simulink model "observer_simulacao_2014a"  (R2014a)
settings: Solver=ode4  StartTime=0.0  StopTime=300  FixedStep=0.1  RelTol=1e-3
settings Model: Creator=icaro  LastModifiedBy=MatheusWhite
settings DebuggingCC: MergeDetectMultiDrivingBlocksExec=error  FrameProcessingCompatibilityMsg=error

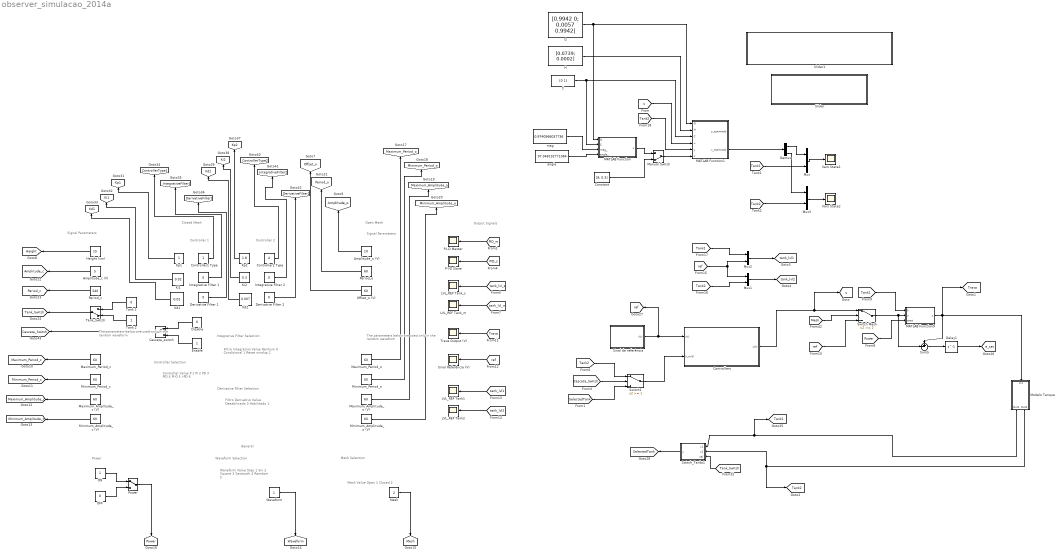
== system observer_simulacao_2014a ==
  note: Waveform Selection
  note: Mesh Selection
  note: Signal Parameters
  note: The parameters below are used only in the random waveform
  note: Filtro Integrativo
      | Value
      |
      | Nenhum
      | 0
      |
      | Condicional
      | 1
      |
      | Reset windup
      | 2
  note: Power
  note: Controller
      | Value
      |
      | P
      | 1
      |
      | PI
      | 2
      |
      | PD
      | 3
      |
      | PID
      | 4
      |
      | PI-D
      | 5
      |
      | I-PD
      | 6
  note: General
  note: Derivative Filter Selection
  note: Closed Mesh
  note: The parameters below are used only in the random waveform
  note: Signal Parameters
  note: Controller 2
  note: Mesh
      | Value
      |
      | Open
      | 1
      |
      | Closed
      | 2
  note: Filtro Derivativo
      | Value
      |
      | Desabilitado
      | 0
      |
      | Habilitado
      | 1
  note: Waveform
      | Value
      |
      | Step
      | 1
      |
      | Sin
      | 2
      |
      | Square
      | 3
      |
      | Sawtooth
      | 4
      |
      | Ramdom
      | 5
  note: Open Mesh
  note: Output Signals
  note: Integrative Filter Selection
  note: Controller 1
  note: Controller Selection
  Amplitude_c (V) : Constant  Value=5
  Amplitude_o (V) : Constant  Value=10
  C : Constant  Value=[0 1]  VectorParams1D=off
  Cascata_switch : ManualSwitch
  Constant : Constant  Value=[8; 0.3]
  Controller1 Type : Constant
  Controller2 Type : Constant  Value=4
  Controllers : Subsystem
  Delay1 : Delay  DelayLength=1  InitialCondition=0
  Demux : Demux  Outputs=2
  Derivative Filter 1 : Constant  Value=0
  Derivative Filter 2 : Constant  Value=0
  Disable : Constant  Value=0
  Enable : Constant
  G : Constant  Value=[0.9942 0; 0.0057 0.9942]  VectorParams1D=off
  H : Constant  Value=[0.0739; 0.0002]  VectorParams1D=off
  Height (cm) : Constant  Value=15
  Integrative Filter 1 : Constant  Value=0
  Integrative Filter 2 : Constant  Value=0
  Kd1 : Constant  Value=0.01
  Kd2 : Constant  Value=0.007
  Ki1 : Constant  Value=0.02
  Ki2 : Constant  Value=0.3
  Kp1 : Constant
  Kp2 : Constant  Value=1.8
  LVL_REF Tank1 : Scope
      settings: TimeRange=100  ShowLegends=on  MaxDataPoints=5000  SaveName=tank1level1  YMin=0  YMax=30  SampleTime=-1  DataFormat=Array
  LVL_REF Tank2 : Scope
      settings: TimeRange=250  ShowLegends=on  MaxDataPoints=5000  SaveName=tank2level1  YMin=0  YMax=30  SampleTime=-1  DataFormat=Array
  "LVL_REF Tank_m " : Scope
      settings: TimeRange=300  ShowLegends=on  MaxDataPoints=5000  SaveName=tank2level  YMin=0  YMax=30  SampleTime=-1  DataFormat=Array
  LVL_REF Tank_s : Scope
      settings: TimeRange=300  ShowLegends=on  MaxDataPoints=5000  SaveName=tank1level  YMin=-90  YMax=130  SampleTime=-1  DataFormat=Array
  MATLAB Function : MATLAB Function  TreatAsAtomicUnit=on
      settings: PermitHierarchicalResolution=ParametersOnly
  MATLAB Function1 : MATLAB Function  TreatAsAtomicUnit=on
      settings: PermitHierarchicalResolution=ParametersOnly
  MATLAB Function9 : MATLAB Function  TreatAsAtomicUnit=on
      settings: PermitHierarchicalResolution=ParametersOnly
  Manual Switch : ManualSwitch  CurrentSetting=0
  Maximum_Amplitude_c (V) : Constant  Value=60
  Maximum_Amplitude_o (V) : Constant  Value=60
  Maximum_Period_c : Constant  Value=60
  Maximum_Period_o : Constant  Value=60
  Mesh : Constant  Value=2
  Minimum_Amplitude_c (V) : Constant  Value=60
  Minimum_Amplitude_o (V) : Constant  Value=60
  Minimum_Period_c : Constant  Value=60
  Minimum_Period_o : Constant  Value=60
  Modelo Tanque : Subsystem
  Mux{,1..3} (4 alike) : Mux  Inputs=2
  OFF : Constant  Value=0
  ON : Constant
  Offset_o (V) : Constant  Value=60
  P-I-D Master : Scope
      settings: TimeRange=300  ShowLegends=on  MaxDataPoints=5000  SaveName=PID1  YMin=-35  YMax=30  SampleTime=-1  DataFormat=Array
  P-I-D Slave : Scope
      settings: TimeRange=300  ShowLegends=on  MaxDataPoints=5000  SaveName=PID2  YMin=-35  YMax=80  SampleTime=-1  DataFormat=Array
  Period_c : Constant  Value=240
  Period_o : Constant  Value=60
  Power : ManualSwitch
  Sinal Referência (V) : Scope
      settings: TimeRange=300  MaxDataPoints=5000  SaveName=meshoutput  YMin=0  YMax=30  SampleTime=-1  DataFormat=Array
  Sinal de referência : Subsystem
  Slider : Subsystem  Description=Replaced Block  mask(Replaced Block){}
      mask help: This block has been replaced with an empty subsystem because it used functionality that is unavailable in Simulink R2014a.
      mask Display: fprintf('Replaced: %s\n','Dashboard Widget')
  Slider1 : Subsystem  Description=Replaced Block  mask(Replaced Block){}
      mask help: This block has been replaced with an empty subsystem because it used functionality that is unavailable in Simulink R2014a.
      mask Display: fprintf('Replaced: %s\n','Dashboard Widget')
  Sum5 : Sum  Inputs=+-|
  Switch Mesh : Switch  Threshold=2
  Switch1 : Switch  Threshold=1
  Switch_Tanks1 : MATLAB Function  TreatAsAtomicUnit=on
      settings: PermitHierarchicalResolution=ParametersOnly
  Tank 1 : Constant  Value=0
  Tank 2 : Constant
  Tank_Switch : ManualSwitch  CurrentSetting=0
  Trava Output (V) : Scope
      settings: TimeRange=300  MaxDataPoints=5000  SaveName=meshoutput2  YMin=-4.5  YMax=4.5  SampleTime=-1  DataFormat=Array
  Vars State1 : Scope
      settings: TimeRange=300  ShowLegends=on  MaxDataPoints=5000  SaveToWorkspace=off  SaveName=ScopeData  YMin=-1.00000  YMax=30.00000  SampleTime=-1
  Vars State2 : Scope
      settings: TimeRange=300  ShowLegends=on  MaxDataPoints=5000  SaveToWorkspace=off  YMin=-1.85008  YMax=16.65074  SampleTime=-1
  Waveform : Constant
  angle : Constant  Value=97.048192771084
  mag : Constant  Value=0.9740566037736
  tag scope: Amplitude_c=global, Amplitude_o=global, Cascata_Switch=global, ControllerType1=global, ControllerType2=global, DerivativeFilter1=global, DerivativeFilter2=global, Height=global, IntegrativeFilter1=global, IntegrativeFilter2=global, Kd1=global, Kd2=global, Ki1=global, Ki2=global, Kp1=global, Kp2=global, Maximum_Amplitude_c=global, Maximum_Amplitude_o=global, Maximum_Period_c=global, Maximum_Period_o=global, Mesh=global, Minimum_Amplitude_c=global, Minimum_Amplitude_o=global, Minimum_Period_c=global, Minimum_Period_o=global, Offset_o=global, Period_c=global, Period_o=global, Power=global, SelectedTank=global, Tank1=global, Tank2=global, Tank_Switch=global, Trava=global, Waveform=global, e_sat=global, ref=global, tank_lvl1=global, tank_lvl2=global, u=global
  wires:
  Maximum_Period_o/1 -> [Maximum_Period_o]
  Integrative Filter 2/1 -> [IntegrativeFilter2]
  [Power] -> MATLAB Function9/3(start)
  MATLAB Function/1(L) -> Manual Switch/1
  Manual Switch/1 -> MATLAB Function1/6(L)
  Controller2 Type/1 -> [ControllerType2]
  [Tank1] -> Mux/2
  [tank_lvl_m] -> "LVL_REF Tank_m "/1
  Switch_Tanks1/1(y) -> [SelectedTank]
  [Tank2] -> MATLAB Function1/5(y)
  [ref] -> Mux2/2, Mux1/1
  Minimum_Amplitude_o (V)/1 -> [Minimum_Amplitude_o]
  [Tank2] -> Mux1/2
  Minimum_Period_o/1 -> [Minimum_Period_o]
  MATLAB Function1/2(x_estimado) -> Demux/1
  [Tank_Switch] -> Switch_Tanks1/3(sel)
  [tank_lvl2] -> LVL_REF Tank2/1
  Mux/1 -> Vars State1/1
  Amplitude_o (V)/1 -> [Amplitude_o]
  [PID_m] -> P-I-D Master/1
  Mux1/1 -> [tank_lvl2]
  Delay1/1 -> [e_sat]
  angle/1 -> MATLAB Function/4(angle_)
  mag/1 -> MATLAB Function/3(mag_)
  Power/1 -> [Power]
  [Trava] -> Trava Output (V)/1
  Disable/1 -> Cascata_switch/1
  [ref] -> Switch Mesh/3
  Kp2/1 -> [Kp2]
  [Tank1] -> MATLAB Function9/1(h)
  Controllers/1(u(t)) -> [u], Switch Mesh/1
  [Tank1] -> Mux2/1
  Sinal de referência/1(r(t)) -> Controllers/1(r(t)), [ref]
  Minimum_Amplitude_c (V)/1 -> [Minimum_Amplitude_c]
  [tank_lvl1] -> LVL_REF Tank1/1
  [Mesh] -> Switch Mesh/2
  Sum5/1 -> Delay1/1
  Modelo Tanque/1(Out1) -> Switch_Tanks1/1(x1), [Tank1]
  Derivative Filter 2/1 -> [DerivativeFilter2]
  Switch Mesh/1 -> Sum5/2, MATLAB Function9/2(u)
  Integrative Filter 1/1 -> [IntegrativeFilter1]
  Enable/1 -> Cascata_switch/2
  Cascata_switch/1 -> [Cascata_Switch]
  [u] -> MATLAB Function1/4(u)
  Controller1 Type/1 -> [ControllerType1]
  Period_o/1 -> [Period_o]
  [ref] -> Sinal Referência (V)/1
  Tank 1/1 -> Tank_Switch/1
  [Cascata_Switch] -> Switch1/2
  Kd2/1 -> [Kd2]
  Kd1/1 -> [Kd1]
  Ki2/1 -> [Ki2]
  Amplitude_c (V)/1 -> [Amplitude_c]
  Height (cm)/1 -> [Height]
  OFF/1 -> Power/2
  [tank_lvl_s] -> LVL_REF Tank_s/1
  [PID_s] -> P-I-D Slave/1
  [SelectedTank] -> Switch1/3
  Minimum_Period_c/1 -> [Minimum_Period_c]
  Period_c/1 -> [Period_c]
  Maximum_Period_c/1 -> [Maximum_Period_c]
  Tank 2/1 -> Tank_Switch/2
  Ki1/1 -> [Ki1]
  Maximum_Amplitude_o (V)/1 -> [Maximum_Amplitude_o]
  Offset_o (V)/1 -> [Offset_o]
  Waveform/1 -> [Waveform]
  Kp1/1 -> [Kp1]
  Constant/1 -> Manual Switch/2
  Maximum_Amplitude_c (V)/1 -> [Maximum_Amplitude_c]
  MATLAB Function9/1(y) -> Modelo Tanque/1(In1), [Trava], Sum5/1
  Tank_Switch/1 -> [Tank_Switch]
  Modelo Tanque/2(Out2) -> Switch_Tanks1/2(x2), [Tank2]
  [Tank2] -> Switch1/1
  Mux2/1 -> [tank_lvl1]
  Derivative Filter 1/1 -> [DerivativeFilter1]
  ON/1 -> Power/1
  Mesh/1 -> [Mesh]
  Switch1/1 -> Controllers/2(h_m(t))
  Demux/1 -> Mux/1
  Mux3/1 -> Vars State2/1
  [Tank2] -> Mux3/2
  Demux/2 -> Mux3/1
  C/1 -> MATLAB Function1/3(C), MATLAB Function/2(C)
  G/1 -> MATLAB Function1/1(G), MATLAB Function/1(G)
  H/1 -> MATLAB Function1/2(H)

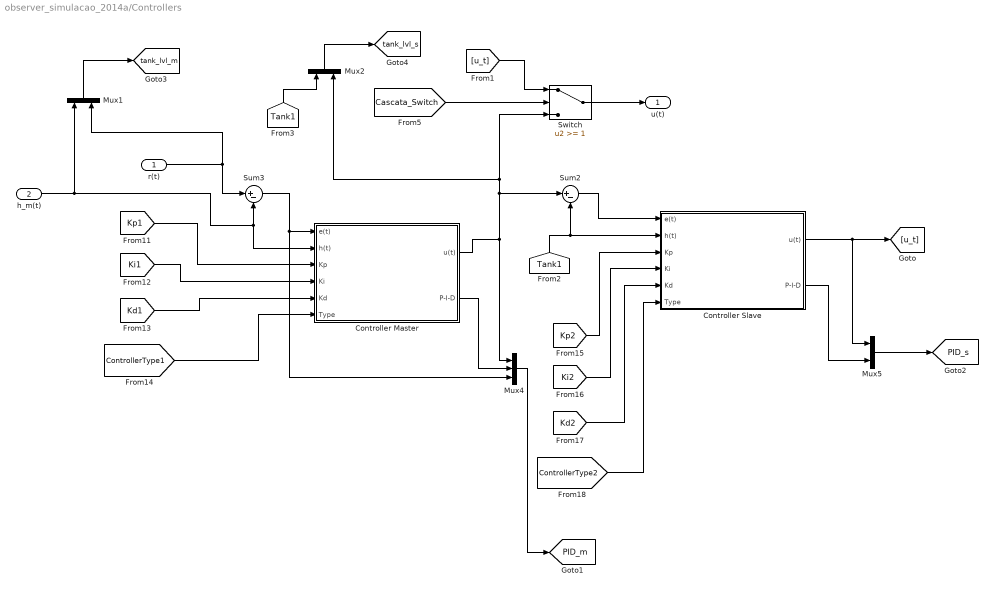
== system observer_simulacao_2014a/Controllers ==
  r(t) : Inport
  h_m(t) : Inport  Port=2
  Controller Master : Subsystem
  Controller Slave : Subsystem
  Mux1 : Mux  Inputs=2
  Mux2 : Mux  Inputs=2
  Mux4 : Mux  Inputs=3
  Mux5 : Mux  Inputs=2
  Sum2 : Sum  Inputs=|+-
  Sum3 : Sum  Inputs=|+-
  Switch : Switch  Threshold=1
  u(t) : Outport
  tag scope: PID_m=global, PID_s=global, tank_lvl_m=global, tank_lvl_s=global
  wires:
  [Tank1] -> Controller Slave/2(h(t)), Sum2/2
  [Kd1] -> Controller Master/5(Kd)
  Controller Slave/2(P-I-D) -> Mux5/2
  [Kp2] -> Controller Slave/3(Kp)
  [Ki2] -> Controller Slave/4(Ki)
  [Ki1] -> Controller Master/4(Ki)
  [Kd2] -> Controller Slave/5(Kd)
  [ControllerType2] -> Controller Slave/6(Type)
  [Kp1] -> Controller Master/3(Kp)
  [ControllerType1] -> Controller Master/6(Type)
  h_m(t)/1 -> Sum3/2, Controller Master/2(h(t)), Mux1/1
  Controller Master/1(u(t)) -> Mux2/2, Switch/3, Sum2/1, Mux4/1
  Sum2/1 -> Controller Slave/1(e(t))
  Controller Slave/1(u(t)) -> [u_t], Mux5/1
  r(t)/1 -> Sum3/1, Mux1/2
  Switch/1 -> u(t)/1
  [Cascata_Switch] -> Switch/2
  Sum3/1 -> Mux4/3, Controller Master/1(e(t))
  [u_t] -> Switch/1
  Mux1/1 -> [tank_lvl_m]
  [Tank1] -> Mux2/1
  Mux2/1 -> [tank_lvl_s]
  Mux4/1 -> [PID_m]
  Mux5/1 -> [PID_s]
  Controller Master/2(P-I-D) -> Mux4/2

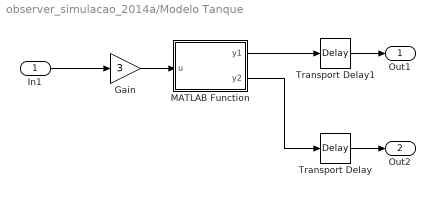
== system observer_simulacao_2014a/Modelo Tanque ==
  In1 : Inport
  Gain : Gain  Gain=3
  MATLAB Function : MATLAB Function  TreatAsAtomicUnit=on
      settings: PermitHierarchicalResolution=ParametersOnly
  Transport Delay : TransportDelay  DelayTime=2
  Transport Delay1 : TransportDelay  DelayTime=2
  Out1 : Outport
  Out2 : Outport  Port=2
  wires:
  Gain/1 -> MATLAB Function/1(u)
  Transport Delay/1 -> Out2/1
  Transport Delay1/1 -> Out1/1
  MATLAB Function/1(y1) -> Transport Delay1/1
  MATLAB Function/2(y2) -> Transport Delay/1
  In1/1 -> Gain/1

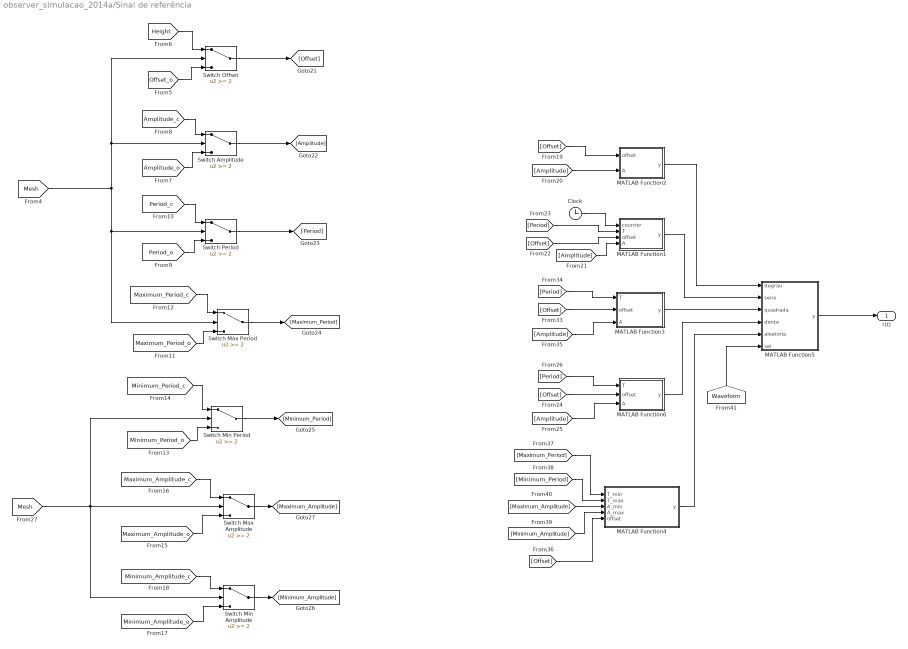
== system observer_simulacao_2014a/Sinal de referência ==
  Clock : Clock
  MATLAB Function1 : MATLAB Function  TreatAsAtomicUnit=on
      settings: PermitHierarchicalResolution=ParametersOnly
  MATLAB Function2 : MATLAB Function  TreatAsAtomicUnit=on
      settings: PermitHierarchicalResolution=ParametersOnly
  MATLAB Function3 : MATLAB Function  TreatAsAtomicUnit=on
      settings: PermitHierarchicalResolution=ParametersOnly
  MATLAB Function4 : MATLAB Function  TreatAsAtomicUnit=on
      settings: PermitHierarchicalResolution=ParametersOnly
  MATLAB Function5 : MATLAB Function  TreatAsAtomicUnit=on
      settings: PermitHierarchicalResolution=ParametersOnly
  MATLAB Function6 : MATLAB Function  TreatAsAtomicUnit=on
      settings: PermitHierarchicalResolution=ParametersOnly
  Switch Amplitude : Switch  Threshold=2
  Switch Max Amplitude : Switch  Threshold=2
  Switch Max Period : Switch  Threshold=2
  Switch Min Amplitude : Switch  Threshold=2
  Switch Min Period : Switch  Threshold=2
  Switch Offset : Switch  Threshold=2
  Switch Period : Switch  Threshold=2
  r(t) : Outport
  wires:
  Clock/1 -> MATLAB Function1/1(counter)
  MATLAB Function5/1(y) -> r(t)/1
  [Mesh] -> Switch Max Period/2, Switch Period/2, Switch Offset/2, Switch Amplitude/2
  [Offset] -> MATLAB Function6/2(offset)
  Switch Min Amplitude/1 -> [Minimum_Amplitude]
  [Period] -> MATLAB Function6/1(T)
  Switch Amplitude/1 -> [Amplitude]
  Switch Period/1 -> [Period]
  Switch Offset/1 -> [Offset]
  [Amplitude] -> MATLAB Function2/2(A)
  Switch Min Period/1 -> [Minimum_Period]
  [Amplitude] -> MATLAB Function1/4(A)
  Switch Max Amplitude/1 -> [Maximum_Amplitude]
  Switch Max Period/1 -> [Maximum_Period]
  [Offset] -> MATLAB Function1/3(offset)
  [Offset] -> MATLAB Function2/1(offset)
  [Period] -> MATLAB Function1/2(T)
  [Amplitude] -> MATLAB Function6/3(A)
  [Period] -> MATLAB Function3/1(T)
  MATLAB Function1/1(y) -> MATLAB Function5/2(seno)
  [Waveform] -> MATLAB Function5/6(sel)
  [Maximum_Period] -> MATLAB Function4/1(T_min)
  [Mesh] -> Switch Min Amplitude/2, Switch Max Amplitude/2, Switch Min Period/2
  MATLAB Function2/1(y) -> MATLAB Function5/1(degrau)
  [Maximum_Amplitude] -> MATLAB Function4/3(A_min)
  MATLAB Function6/1(y) -> MATLAB Function5/4(dente)
  [Amplitude] -> MATLAB Function3/3(A)
  [Minimum_Amplitude] -> MATLAB Function4/4(A_max)
  [Offset] -> MATLAB Function4/5(offset)
  MATLAB Function4/1(y) -> MATLAB Function5/5(aleatoria)
  MATLAB Function3/1(y) -> MATLAB Function5/3(quadrada)
  [Offset] -> MATLAB Function3/2(offset)
  [Minimum_Period] -> MATLAB Function4/2(T_max)
  [Offset_o] -> Switch Offset/3
  [Height] -> Switch Offset/1
  [Amplitude_o] -> Switch Amplitude/3
  [Amplitude_c] -> Switch Amplitude/1
  [Period_o] -> Switch Period/3
  [Period_c] -> Switch Period/1
  [Maximum_Period_o] -> Switch Max Period/3
  [Maximum_Period_c] -> Switch Max Period/1
  [Minimum_Period_c] -> Switch Min Period/1
  [Minimum_Period_o] -> Switch Min Period/3
  [Maximum_Amplitude_c] -> Switch Max Amplitude/1
  [Maximum_Amplitude_o] -> Switch Max Amplitude/3
  [Minimum_Amplitude_c] -> Switch Min Amplitude/1
  [Minimum_Amplitude_o] -> Switch Min Amplitude/3

== system observer_simulacao_2014a/Slider ==

== system observer_simulacao_2014a/Slider1 ==

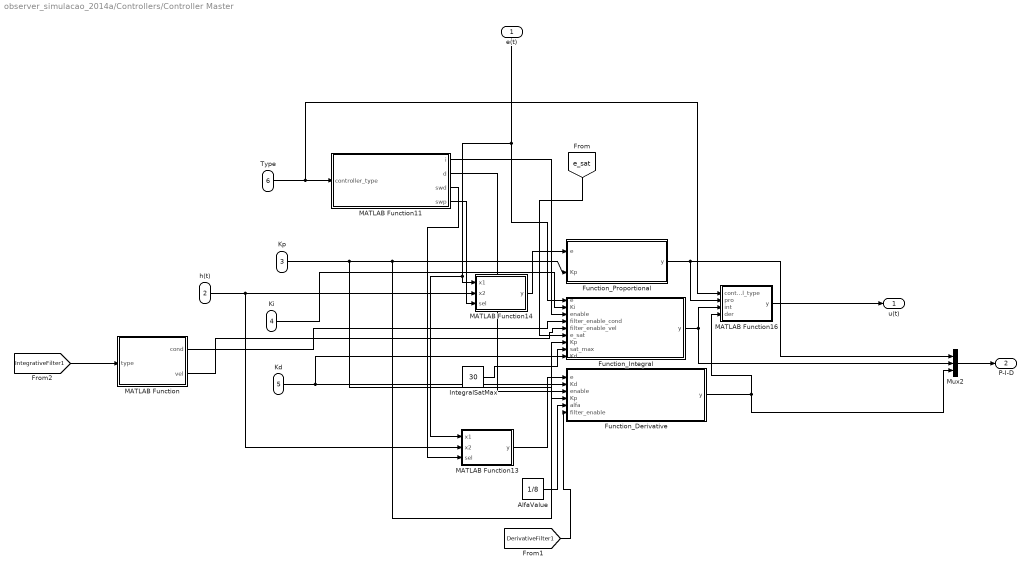
== system observer_simulacao_2014a/Controllers/Controller Master ==
  e(t) : Inport
  h(t) : Inport  Port=2
  Kp : Inport  Port=3
  Ki : Inport  Port=4
  Kd : Inport  Port=5
  Type : Inport  Port=6
  AlfaValue : Constant  Value=1/8
  Function_Derivative : MATLAB Function  TreatAsAtomicUnit=on
      settings: PermitHierarchicalResolution=ParametersOnly
  Function_Integral : MATLAB Function  TreatAsAtomicUnit=on
      settings: PermitHierarchicalResolution=ParametersOnly
  Function_Proportional : MATLAB Function  TreatAsAtomicUnit=on
      settings: PermitHierarchicalResolution=ParametersOnly
  IntegralSatMax : Constant  Value=30
  MATLAB Function : MATLAB Function  TreatAsAtomicUnit=on
      settings: PermitHierarchicalResolution=ParametersOnly
  MATLAB Function11 : MATLAB Function  TreatAsAtomicUnit=on
      settings: PermitHierarchicalResolution=ParametersOnly
  MATLAB Function13 : MATLAB Function  TreatAsAtomicUnit=on
      settings: PermitHierarchicalResolution=ParametersOnly
  MATLAB Function14 : MATLAB Function  TreatAsAtomicUnit=on
      settings: PermitHierarchicalResolution=ParametersOnly
  MATLAB Function16 : MATLAB Function  TreatAsAtomicUnit=on
      settings: PermitHierarchicalResolution=ParametersOnly
  Mux2 : Mux  Inputs=3
  u(t) : Outport
  P-I-D : Outport  Port=2
  wires:
  h(t)/1 -> MATLAB Function13/2(x2), MATLAB Function14/2(x2)
  e(t)/1 -> MATLAB Function13/1(x1), MATLAB Function14/1(x1), Function_Integral/1(e)
  Function_Integral/1(y) -> MATLAB Function16/3(int), Mux2/2
  Kp/1 -> Function_Derivative/4(Kp), Function_Integral/7(Kp), Function_Proportional/2(Kp)
  MATLAB Function11/2(d) -> Function_Derivative/3(enable)
  Function_Proportional/1(y) -> MATLAB Function16/2(pro), Mux2/1
  MATLAB Function11/1(i) -> Function_Integral/3(enable)
  Type/1 -> MATLAB Function16/1(control_type), MATLAB Function11/1(controller_type)
  MATLAB Function11/4(swp) -> MATLAB Function14/3(sel)
  Ki/1 -> Function_Integral/2(Ki)
  MATLAB Function/2(vel) -> Function_Integral/5(filter_enable_vel)
  MATLAB Function11/3(swd) -> MATLAB Function13/3(sel)
  MATLAB Function/1(cond) -> Function_Integral/4(filter_enable_cond)
  IntegralSatMax/1 -> Function_Integral/8(sat_max)
  MATLAB Function14/1(y) -> Function_Proportional/1(e)
  AlfaValue/1 -> Function_Derivative/5(alfa)
  [DerivativeFilter1] -> Function_Derivative/6(filter_enable)
  Function_Derivative/1(y) -> MATLAB Function16/4(der), Mux2/3
  MATLAB Function13/1(y) -> Function_Derivative/1(e)
  Kd/1 -> Function_Integral/9(Kd), Function_Derivative/2(Kd)
  Mux2/1 -> P-I-D/1
  MATLAB Function16/1(y) -> u(t)/1
  [e_sat] -> Function_Integral/6(e_sat)
  [IntegrativeFilter1] -> MATLAB Function/1(type)

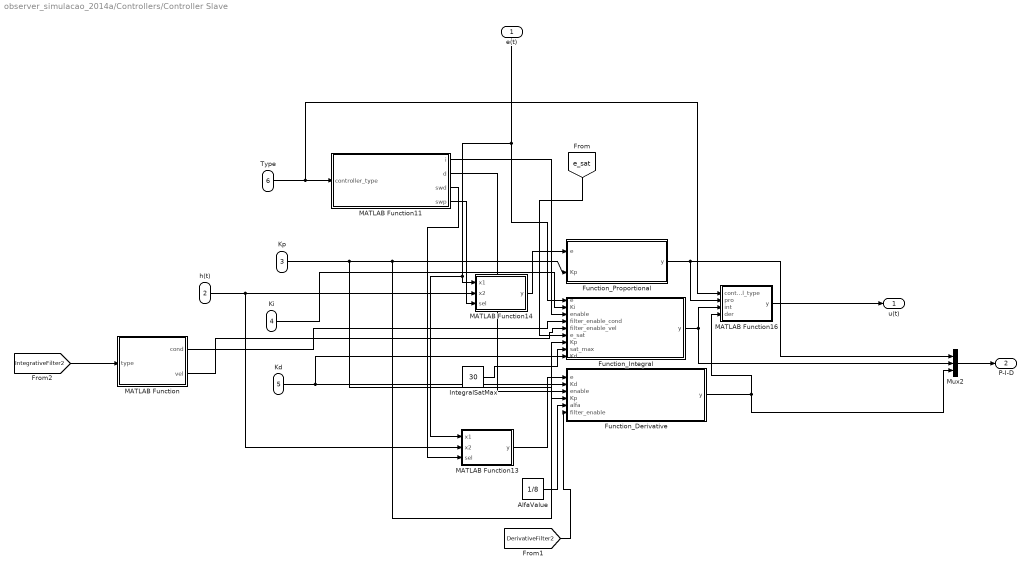
== system observer_simulacao_2014a/Controllers/Controller Slave ==
  e(t) : Inport
  h(t) : Inport  Port=2
  Kp : Inport  Port=3
  Ki : Inport  Port=4
  Kd : Inport  Port=5
  Type : Inport  Port=6
  AlfaValue : Constant  Value=1/8
  Function_Derivative : MATLAB Function  TreatAsAtomicUnit=on
      settings: PermitHierarchicalResolution=ParametersOnly
  Function_Integral : MATLAB Function  TreatAsAtomicUnit=on
      settings: PermitHierarchicalResolution=ParametersOnly
  Function_Proportional : MATLAB Function  TreatAsAtomicUnit=on
      settings: PermitHierarchicalResolution=ParametersOnly
  IntegralSatMax : Constant  Value=30
  MATLAB Function : MATLAB Function  TreatAsAtomicUnit=on
      settings: PermitHierarchicalResolution=ParametersOnly
  MATLAB Function11 : MATLAB Function  TreatAsAtomicUnit=on
      settings: PermitHierarchicalResolution=ParametersOnly
  MATLAB Function13 : MATLAB Function  TreatAsAtomicUnit=on
      settings: PermitHierarchicalResolution=ParametersOnly
  MATLAB Function14 : MATLAB Function  TreatAsAtomicUnit=on
      settings: PermitHierarchicalResolution=ParametersOnly
  MATLAB Function16 : MATLAB Function  TreatAsAtomicUnit=on
      settings: PermitHierarchicalResolution=ParametersOnly
  Mux2 : Mux  Inputs=3
  u(t) : Outport
  P-I-D : Outport  Port=2
  wires:
  h(t)/1 -> MATLAB Function13/2(x2), MATLAB Function14/2(x2)
  e(t)/1 -> MATLAB Function13/1(x1), MATLAB Function14/1(x1), Function_Integral/1(e)
  Function_Integral/1(y) -> MATLAB Function16/3(int), Mux2/2
  Kp/1 -> Function_Derivative/4(Kp), Function_Integral/7(Kp), Function_Proportional/2(Kp)
  MATLAB Function11/2(d) -> Function_Derivative/3(enable)
  Function_Proportional/1(y) -> MATLAB Function16/2(pro), Mux2/1
  MATLAB Function11/1(i) -> Function_Integral/3(enable)
  Type/1 -> MATLAB Function16/1(control_type), MATLAB Function11/1(controller_type)
  MATLAB Function11/4(swp) -> MATLAB Function14/3(sel)
  Ki/1 -> Function_Integral/2(Ki)
  MATLAB Function/2(vel) -> Function_Integral/5(filter_enable_vel)
  MATLAB Function11/3(swd) -> MATLAB Function13/3(sel)
  MATLAB Function/1(cond) -> Function_Integral/4(filter_enable_cond)
  IntegralSatMax/1 -> Function_Integral/8(sat_max)
  MATLAB Function14/1(y) -> Function_Proportional/1(e)
  AlfaValue/1 -> Function_Derivative/5(alfa)
  [DerivativeFilter2] -> Function_Derivative/6(filter_enable)
  Function_Derivative/1(y) -> MATLAB Function16/4(der), Mux2/3
  MATLAB Function13/1(y) -> Function_Derivative/1(e)
  Kd/1 -> Function_Integral/9(Kd), Function_Derivative/2(Kd)
  Mux2/1 -> P-I-D/1
  MATLAB Function16/1(y) -> u(t)/1
  [e_sat] -> Function_Integral/6(e_sat)
  [IntegrativeFilter2] -> MATLAB Function/1(type)

== matlab function observer_simulacao_2014a/Controllers/Controller Slave/Function_Derivative ==
  settings: updateMethod=DISCRETE  sampleTime=0.1
  data: e input; y output; Kd input; enable input; Kp input; alfa input; filter_enable input
function y = derivative(e, Kd, enable, Kp, alfa, filter_enable)

persistent prev_error;
persistent y_error;
persistent aux;

if isempty(prev_error)
   prev_error = 0; 
end

if isempty(y_error)
   y_error = 0; 
end

if isempty(aux)
   aux = 0; 
end


%1/0.1 == 10
Td = Kd/Kp;


if(filter_enable == 1)
    y = ((e - prev_error + alfa*y_error) * Kd)/(1+(Td*alfa));
else
    y = Kd*(e - prev_error)*enable/0.1;
end


prev_error = e;
y_error = y;

end

== matlab function observer_simulacao_2014a/Controllers/Controller Master/MATLAB Function ==
  data: type input; cond output; vel output
function [cond, vel] = IntSwitch(type)

if type == 0
   cond = 0;
   vel = 0;
elseif type == 1
    cond = 1;
    vel = 0;
else
   cond = 0;
   vel = 1;
end

== matlab function observer_simulacao_2014a/Controllers/Controller Slave/Function_Integral ==
  settings: updateMethod=DISCRETE  sampleTime=0.1
  data: e input; y output; Ki input; enable input; filter_enable_cond input; filter_enable_vel input; e_sat input; Kp input; sat_max input; Kd input
function y = integral(e, Ki, enable, filter_enable_cond, filter_enable_vel, e_sat, Kp, sat_max, Kd)

persistent sum;

if isempty(sum)
   sum = 0; 
end

Ti = Kp/Ki;
Td = Kd/Kp;

Tt = sqrt(Ti * Td);

Tt_value = (1/Tt) * e_sat;

if(filter_enable_cond == 1 && sum > sat_max) 
    sum = 0;
elseif(filter_enable_vel == 1)
    sum =  ((Ki*e) + Tt_value)*0.1 + sum;
else
    sum = sum + Ki*e*0.1;
end
y = sum*enable;

== matlab function observer_simulacao_2014a/Controllers/Controller Slave/Function_Proportional ==
  data: e input; y output; Kp input
function y = proportional(e, Kp)

y = Kp*e;

== matlab function observer_simulacao_2014a/Controllers/Controller Slave/MATLAB Function ==
  data: type input; cond output; vel output
function [cond, vel] = IntSwitch(type)

if type == 0
   cond = 0;
   vel = 0;
elseif type == 1
    cond = 1;
    vel = 0;
else
   cond = 0;
   vel = 1;
end

== matlab function observer_simulacao_2014a/Controllers/Controller Slave/MATLAB Function11 ==
  data: controller_type input; i output; d output; swd output; swp output
function [i,d,swd,swp]= fcn(controller_type)

if(controller_type == 1)
    i = 0;
    d = 0;
    swd = 0;
    swp = 0;
elseif(controller_type == 2)
    i = 1;
    d = 0;
    swd = 0;
    swp = 0;
elseif(controller_type == 3)
    i = 0;
    d = 1;
    swd = 0;
    swp = 0;
elseif(controller_type == 4)
    i = 1;
    d = 1;
    swd = 0;
    swp = 0;
elseif(controller_type == 5)
    i = 1;
    d = 1;
    swd = 1;
    swp = 0;
elseif(controller_type == 6)
    i = 1;
    d = 1;
    swd = 1;
    swp = 1;
else
    i = 0;
    d = 0;
    swd = 0;
    swp = 0;
end

== matlab function observer_simulacao_2014a/Controllers/Controller Slave/MATLAB Function13 ==
  data: x1 input; x2 input; y output; sel input
function y = switch_deriv(x1, x2, sel)

if sel == 0
    y = x1; 
else
    y = x2;
end
    
end

== matlab function observer_simulacao_2014a/Controllers/Controller Master/Function_Proportional ==
  data: e input; y output; Kp input
function y = proportional(e, Kp)

y = Kp*e;

== matlab function observer_simulacao_2014a/Controllers/Controller Slave/MATLAB Function14 ==
  data: x1 input; x2 input; y output; sel input
function y = switch_prop(x1, x2, sel)

if sel == 0
    y = x1; 
else
    y = x2;
end
    
end

== matlab function observer_simulacao_2014a/Controllers/Controller Master/Function_Integral ==
  settings: updateMethod=DISCRETE  sampleTime=0.1
  data: e input; y output; Ki input; enable input; filter_enable_cond input; filter_enable_vel input; e_sat input; Kp input; sat_max input; Kd input
function y = integral(e, Ki, enable, filter_enable_cond, filter_enable_vel, e_sat, Kp, sat_max, Kd)

persistent sum;

if isempty(sum)
   sum = 0; 
end

Ti = Kp/Ki;
Td = Kd/Kp;

Tt = sqrt(Ti * Td);

Tt_value = (1/Tt) * e_sat;

if(filter_enable_cond == 1 && sum > sat_max) 
    sum = 0;
elseif(filter_enable_vel == 1)
    sum =  ((Ki*e) + Tt_value)*0.1 + sum;
else
    sum = sum + Ki*e*0.1;
end
y = sum*enable;

== matlab function observer_simulacao_2014a/Controllers/Controller Master/Function_Derivative ==
  settings: updateMethod=DISCRETE
  data: e input; y output; Kd input; enable input; Kp input; alfa input; filter_enable input
function y = derivative(e, Kd, enable, Kp, alfa, filter_enable)

persistent prev_error;
persistent y_error;
persistent aux;

if isempty(prev_error)
   prev_error = 0; 
end

if isempty(y_error)
   y_error = 0; 
end

if isempty(aux)
   aux = 0; 
end


%1/0.1 == 10
Td = Kd/Kp;


if(filter_enable == 1)
    y = ((e - prev_error + alfa*y_error)*enable * Kd)/(1+(Td*alfa));
else
    y = Kd*(e - prev_error)*enable/0.1;
end


prev_error = e;
y_error = y;

end

== matlab function observer_simulacao_2014a/Controllers/Controller Master/MATLAB Function11 ==
  data: controller_type input; i output; d output; swd output; swp output
function [i,d,swd,swp]= fcn(controller_type)

if(controller_type == 1)
    i = 0;
    d = 0;
    swd = 0;
    swp = 0;
elseif(controller_type == 2)
    i = 1;
    d = 0;
    swd = 0;
    swp = 0;
elseif(controller_type == 3)
    i = 0;
    d = 1;
    swd = 0;
    swp = 0;
elseif(controller_type == 4)
    i = 1;
    d = 1;
    swd = 0;
    swp = 0;
elseif(controller_type == 5)
    i = 1;
    d = 1;
    swd = 1;
    swp = 0;
elseif(controller_type == 6)
    i = 1;
    d = 1;
    swd = 1;
    swp = 1;
else
    i = 0;
    d = 0;
    swd = 0;
    swp = 0;
end

== matlab function observer_simulacao_2014a/Modelo Tanque/MATLAB Function ==
  settings: updateMethod=DISCRETE  sampleTime=0.1
  data: u input; y1 output; y2 output
function [y1, y2]= fcn(u)

persistent A1
persistent A2
persistent a1
persistent a2
persistent km
persistent g
persistent t
persistent h1
persistent h2

if(isempty(t))
    A1 = pi*(4.445/2)^2;           %Area transversal do tanque 1
    A2 = pi*(4.445/2)^2;           %Area transversal do tanque 2
    a1 = (0.445/2)^2*pi;     %Area transversal da tubulação de saida em t1 
    a2 =(0.445/2)^2*pi;    %Area transversal da tubulação de saida em t2
    km = 3.3;                %Constante do Motor
    g  = 980.665;               %Constante da gravidade
    h1 = 0;
    h2 = 0;
    t = 10^-1;
end

dh1 = ((km*u) - a1*sqrt(2*g*h1))/A1;
h1 = h1 + t*dh1;
if(h1<0)
    h1 = 0;
end
dh2 = (a1*sqrt(2*g*h1) - a2*sqrt(2*g*h2))/A2;
h2 = h2 + t*dh2;
if(h2<0)
    h2 = 0;
end

y1 = h1;
y2 = h2;

end

== matlab function observer_simulacao_2014a/Controllers/Controller Master/MATLAB Function13 ==
  data: x1 input; x2 input; y output; sel input
function y = switch_deriv(x1, x2, sel)

if sel == 0
    y = x1; 
else
    y = x2;
end
    
end

== matlab function observer_simulacao_2014a/Controllers/Controller Master/MATLAB Function14 ==
  data: x1 input; x2 input; y output; sel input
function y = switch_prop(x1, x2, sel)

if sel == 0
    y = x1; 
else
    y = x2;
end
    
end

== matlab function observer_simulacao_2014a/Controllers/Controller Slave/MATLAB Function16 ==
  data: control_type input; y output; pro input; int input; der input
function y = adding(control_type, pro, int, der)
%#codegen

if(control_type >= 1 && control_type <= 4)
   y = pro + int + der;
elseif(control_type == 5)
    y = pro + int - der;
else
    y = int - pro - der;
end

== matlab function observer_simulacao_2014a/Controllers/Controller Master/MATLAB Function16 ==
  data: control_type input; y output; pro input; int input; der input
function y = adding(control_type, pro, int, der)
%#codegen

if(control_type >= 1 && control_type <= 4)
   y = pro + int + der;
elseif(control_type == 5)
    y = pro + int - der;
else
    y = int - pro - der;
end

== matlab function observer_simulacao_2014a/MATLAB Function ==
  data: G input; C input; mag_ input; L output; angle_ input
function L = calc_L(G, C, mag_, angle_)

Wo = [C; C*G];

angle_ = angle_*(pi/180);

p1 = pol2cart(angle_, mag_);
p2 = pol2cart(-angle_, mag_);

a1 = real(-(p1+p2));
a2 = real(p1*p2);

qc = G^2 + a1*G + a2*eye(2);
invWo = inv(Wo);
L = qc*invWo*[0; 1];

end

== matlab function observer_simulacao_2014a/MATLAB Function1 ==
  settings: updateMethod=DISCRETE  sampleTime=0.1
  data: G input; H input; C input; u input; y input; L input; y_estimado output; x_estimado output
function [y_estimado, x_estimado] = observer(G, H, C, u, y, L)

% persistent x_next
% 
% if(isempty(x_next))
%     x_next = [0; 0];
% end
% 
% x_estimado = x_next;
% y_estimado = C*x_estimado;
% x_next = G*x_estimado + H*u + L*(y-y_estimado);

persistent x_hat

if(isempty(x_hat))
    x_hat = [0; y];
end

x_estimado = x_hat;
y_estimado = C*x_hat;

x_hat = G*x_hat + H*u + L*(y-y_estimado);

end

== matlab function observer_simulacao_2014a/MATLAB Function9 ==
  data: h input; u input; y output; start input
    function y = travas(h, u, start)
%#codegen
h_max = 30;

%Trava de tensÃ£o
if(u < -4)
    u = -4;
end
if(u > 4)
    u = 4;
end

%Trava pra nÃ£o sugar ar
if(u < 0 & h < 2)
    u = 0;
end

%Trava de transbordamento
% if(h >= h_max - 1.0 & h < h_max - 0.75)
%    u = 0.95*u;
% elseif(h >= h_max - 0.75 & h < h_max - 0.5)
%     u = 0.93*u;
% elseif(h >= h_max - 0.5 & h < h_max - 0.25)
%     u = 0.91*u;
% elseif(h >= h_max - 0.25 & h < h_max)
%     u = 0.88*u;
% elseif(h >= h_max)
%     u = 0;
% end

%
if h >= (h_max-1)
    u = (h_max - h)*u;
end

%
% persistent goingup
% 
% if isempty(goingup)
%    goingup = 1; 
% end
% 
% if goingup == 1
%    if h >= 29
%       u = 0;
%       goingup = 0;
%    end
% else
%     if h <= 25
%        goingup = 1; 
%     else
%        u = 0; 
%     end
% end
    
y = start*u;

== matlab function observer_simulacao_2014a/Sinal de referência/MATLAB Function1 ==
  data: counter input; y output; T input; offset input; A input
function y = seno(counter, T, offset, A)

%counter = cast(counter, 'double');

y = A*sin(counter*2*pi/T) + offset;

== matlab function observer_simulacao_2014a/Sinal de referência/MATLAB Function2 ==
  data: offset input; y output; A input
function y = degrau(offset, A)

y = offset;

== matlab function observer_simulacao_2014a/Sinal de referência/MATLAB Function3 ==
  data: y output; T input; offset input; A input
function y = quadrada(T, offset, A)

persistent counter_q;

if isempty(counter_q)
   counter_q = 0; 
end

counter_q = counter_q + 1;

if (counter_q <= 5*T)
    y = -A + offset;
elseif (counter_q > 5*T)
    y = A + offset;
else
    y = 0;
end

if (counter_q >= 10*T)
   counter_q = 0; 
end

== matlab function observer_simulacao_2014a/Sinal de referência/MATLAB Function4 ==
  data: T_min input; y output; T_max input; A_min input; A_max input; offset input
function y = aleatoria(T_min, T_max, A_min, A_max, offset)

persistent T_now;
persistent A_now;
persistent counter_a;

if isempty(counter_a)
    T_now = T_min + (T_max - T_min)*rand;
    A_now = A_min + (A_max - A_min)*rand + offset;
    counter_a = 0;
end

counter_a = counter_a + 1;

y = A_now;

if (counter_a >= T_now*10)
    T_now = T_min + (T_max - T_min)*rand;
    A_now = A_min + (A_max - A_min)*rand + offset;
    counter_a = 0;
end

== matlab function observer_simulacao_2014a/Sinal de referência/MATLAB Function5 ==
  data: degrau input; y output; seno input; quadrada input; dente input; aleatoria input; sel input
function y = mux(degrau, seno, quadrada, dente, aleatoria, sel)

switch sel
    case 1
        y = degrau;
    case 2
        y = seno;
    case 3
        y = quadrada;
    case 4
        y = dente;
    case 5
        y = aleatoria;
    otherwise
        y = 0;
end

== matlab function observer_simulacao_2014a/Sinal de referência/MATLAB Function6 ==
  data: y output; T input; offset input; A input
function y = dente(T, offset, A)

persistent counter_d;

if isempty(counter_d)
   counter_d = 0; 
end


y = counter_d*A*2/(10*T) + offset - A;

counter_d = counter_d + 1;

if (counter_d > T*10)
   counter_d = 0;
end

== matlab function observer_simulacao_2014a/Switch_Tanks1 ==
  data: x1 input; x2 input; y output; sel input
function y = switch2(x1, x2, sel)

if sel == 0
    y = x1; 
else
    y = x2;
end
    
end
